simulink model "dualArrayTestComplete_noTrigger"  (R2012b)
settings: Solver=FixedStepDiscrete  StartTime=0.0  StopTime=inf  FixedStep=0.001  RelTol=1e-3
settings Model: ExplicitPartitioning=on  Creator=gilja  LastModifiedBy=NPTL
settings SolverCC: EnableConcurrentExecution=on  ConcurrentTasks=on
settings OptimizationCC: InlineParams=on  InlineInvariantSignals=on  EnhancedBackFolding=on  EfficientFloat2IntCast=on
settings HardwareCC: ProdIntDivRoundTo=Zero  ProdEndianess=LittleEndian  ProdHWDeviceType=Generic->32-bit x86 compatible
settings ModelReferenceCC: UpdateModelReferenceTargets=IfOutOfDate  ModelReferenceMinAlgLoopOccurrences=on
settings RTWCC: SystemTargetFile=xpctarget.tlc  TemplateMakefile=xpc_default_tmf  Description=xPC Target  ProcessScript=xpctarget_make_rtw_hook  RTWCompilerOptimization=On
settings CodeAppCC: MaxIdLength=62
settings xpcTargetCC: TargetFcnLib=ansi_tfl_table_tmw.mat  CodeReplacementLibrary=XPC_BLAS  ParMdlRefBuildCompliant=on  ConcurrentExecutionCompliant=on  CombineSignalStateStructs=off  GRTInterface=on  xPCTaskExecutionProfile=on  xPCRL32EventNumber=5000  xPCIRQSourceBoard=Parallel_Port  xPCIOIRQSlot=0x378  xPCisDownloadable=off  xPCLoadParamSetFile=off  xPCConcurrentTasks=off  xPCEnableSFAnimation=off

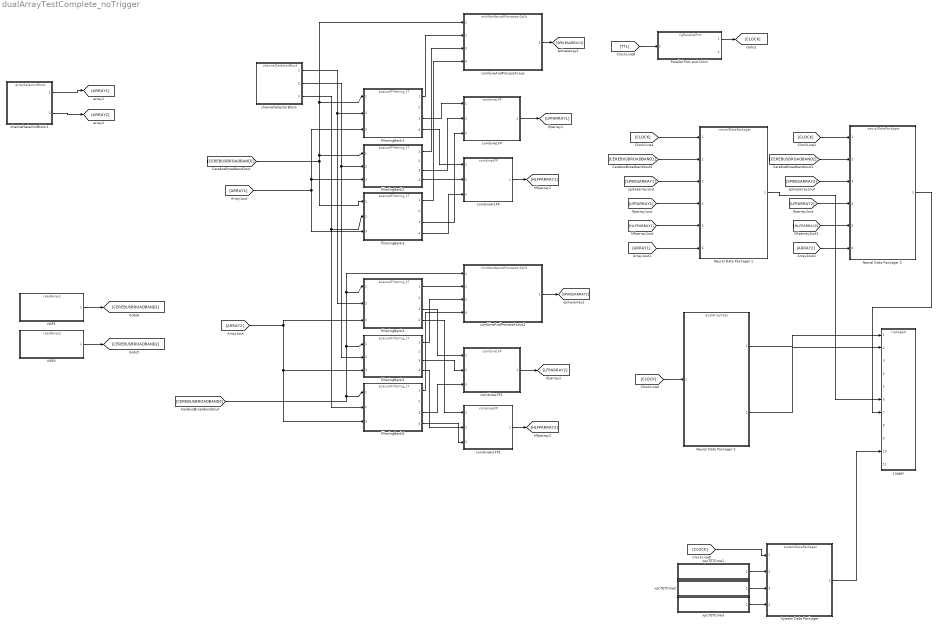
== system dualArrayTestComplete_noTrigger ==
  Logger : ModelReference  ModelNameDialog=rigLogger  SimulationMode=Normal  ModelReferenceVersion=1.134  CopyOfModelName=rigLogger  DefaultDataLogging=on
  NSP1 : ModelReference  ModelNameDialog=readArray1  SimulationMode=Normal  ModelReferenceVersion=1.97  CopyOfModelName=readArray1  DefaultDataLogging=on
  NSP2 : ModelReference  ModelNameDialog=readArray2  SimulationMode=Normal  ModelReferenceVersion=1.98  CopyOfModelName=readArray2  DefaultDataLogging=on
  Neural Data Packager 1 : ModelReference  ModelNameDialog=neuralDataPackager  SimulationMode=Normal  ModelReferenceVersion=1.161  CopyOfModelName=neuralDataPackager  DefaultDataLogging=on
  Neural Data Packager 2 : ModelReference  ModelNameDialog=neuralDataPackager  SimulationMode=Normal  ModelReferenceVersion=1.161  CopyOfModelName=neuralDataPackager  DefaultDataLogging=on
  Neural Data Packager 3 : ModelReference  ModelNameDialog=dualArrayTask  SimulationMode=Normal  ModelReferenceVersion=1.98  CopyOfModelName=dualArrayTask  DefaultDataLogging=on
  Parallel Port and Clock : ModelReference  ModelNameDialog=rigParallelPort  SimulationMode=Normal  ModelReferenceVersion=1.93  CopyOfModelName=rigParallelPort  DefaultDataLogging=on
  System Data Packager : ModelReference  Priority=0  ModelNameDialog=systemDataPackager  SimulationMode=Normal  ModelReferenceVersion=1.180  CopyOfModelName=systemDataPackager  DefaultDataLogging=on
  channelSelectorBlock : ModelReference  ModelNameDialog=channelSelectorBlock  SimulationMode=Normal  ModelReferenceVersion=1.36  CopyOfModelName=channelSelectorBlock  DefaultDataLogging=on
  channelSelectorBlock1 : ModelReference  ModelNameDialog=arraySelectorBlock  SimulationMode=Normal  ModelReferenceVersion=1.40  CopyOfModelName=arraySelectorBlock  DefaultDataLogging=on
  combineAndProcessAcaus : ModelReference  ModelNameDialog=minMaxNeuralProcessorSplit  SimulationMode=Normal  ModelReferenceVersion=1.34  CopyOfModelName=minMaxNeuralProcessorSplit  DefaultDataLogging=on
  combineAndProcessAcaus1 : ModelReference  ModelNameDialog=minMaxNeuralProcessorSplit  SimulationMode=Normal  ModelReferenceVersion=1.34  CopyOfModelName=minMaxNeuralProcessorSplit  DefaultDataLogging=on
  combineHLFP : ModelReference  ModelNameDialog=combineLFP  SimulationMode=Normal  ModelReferenceVersion=1.38  CopyOfModelName=combineLFP  DefaultDataLogging=on
  combineHLFP1 : ModelReference  ModelNameDialog=combineLFP  SimulationMode=Normal  ModelReferenceVersion=1.38  CopyOfModelName=combineLFP  DefaultDataLogging=on
  combineLFP : ModelReference  ModelNameDialog=combineLFP  SimulationMode=Normal  ModelReferenceVersion=1.38  CopyOfModelName=combineLFP  DefaultDataLogging=on
  combineLFP1 : ModelReference  ModelNameDialog=combineLFP  SimulationMode=Normal  ModelReferenceVersion=1.38  CopyOfModelName=combineLFP  DefaultDataLogging=on
  filteringBank{1..6} (6 alike) : ModelReference  ModelNameDialog=acausalFiltering_t7  SimulationMode=Normal  ModelReferenceVersion=1.72  CopyOfModelName=acausalFiltering_t7  DefaultDataLogging=on
  xpcTETCore1 : ModelReference  Priority=0  ModelNameDialog=xpcTETMulticore  SimulationMode=Normal  ModelReferenceVersion=1.188  CopyOfModelName=xpcTETMulticore  DefaultDataLogging=on
  xpcTETCore2 : ModelReference  Priority=0  ModelNameDialog=xpcTETMulticore  SimulationMode=Normal  ModelReferenceVersion=1.188  CopyOfModelName=xpcTETMulticore  DefaultDataLogging=on
  xpcTETCore3 : ModelReference  Priority=0  ModelNameDialog=xpcTETMulticore  SimulationMode=Normal  ModelReferenceVersion=1.188  CopyOfModelName=xpcTETMulticore  DefaultDataLogging=on
  wires:
  filteringBank1/1 -> combineAndProcessAcaus/2
  channelSelectorBlock/1 -> filteringBank4/2, filteringBank1/2
  channelSelectorBlock/2 -> filteringBank5/2, filteringBank2/2
  filteringBank2/1 -> combineAndProcessAcaus/3
  channelSelectorBlock/3 -> filteringBank6/2, filteringBank3/2
  filteringBank3/1 -> combineAndProcessAcaus/4
  filteringBank1/4 -> combineHLFP/1
  filteringBank2/4 -> combineHLFP/2
  filteringBank3/4 -> combineHLFP/3
  [SPIKESARRAY1] -> Neural Data Packager 1/3
  Neural Data Packager 1/1 -> Logger/6
  filteringBank1/3 -> combineLFP/1
  filteringBank2/3 -> combineLFP/2
  filteringBank3/3 -> combineLFP/3
  [CEREBUSBROADBAND1] -> filteringBank3/1, filteringBank2/1, combineAndProcessAcaus/1, filteringBank1/1
  [CEREBUSBROADBAND2] -> filteringBank6/1, filteringBank5/1, filteringBank4/1, combineAndProcessAcaus1/1
  filteringBank4/3 -> combineLFP1/1
  filteringBank5/3 -> combineLFP1/2
  filteringBank5/4 -> combineHLFP1/2
  filteringBank6/3 -> combineLFP1/3
  filteringBank4/4 -> combineHLFP1/1
  filteringBank6/4 -> combineHLFP1/3
  filteringBank4/1 -> combineAndProcessAcaus1/2
  filteringBank5/1 -> combineAndProcessAcaus1/3
  filteringBank6/1 -> combineAndProcessAcaus1/4
  Neural Data Packager 2/1 -> Logger/7
  [ARRAY1] -> filteringBank2/3, filteringBank1/3, filteringBank3/3
  [ARRAY2] -> filteringBank4/3, filteringBank6/3, filteringBank5/3
  Parallel Port and Clock/1 -> [CLOCK]
  [CLOCK] -> Neural Data Packager 2/1
  [CLOCK] -> Neural Data Packager 1/1
  combineHLFP/1 -> [HLFPARRAY1]
  [HLFPARRAY1] -> Neural Data Packager 1/5
  combineHLFP1/1 -> [HLFPARRAY2]
  [HLFPARRAY2] -> Neural Data Packager 2/5
  combineAndProcessAcaus1/1 -> [SPIKESARRAY2]
  [SPIKESARRAY2] -> Neural Data Packager 2/3
  combineAndProcessAcaus/1 -> [SPIKESARRAY1]
  combineLFP/1 -> [LFPARRAY1]
  [LFPARRAY1] -> Neural Data Packager 1/4
  combineLFP1/1 -> [LFPARRAY2]
  [LFPARRAY2] -> Neural Data Packager 2/4
  [CEREBUSBROADBAND1] -> Neural Data Packager 1/2
  [CEREBUSBROADBAND2] -> Neural Data Packager 2/2
  channelSelectorBlock1/1 -> [ARRAY1]
  channelSelectorBlock1/2 -> [ARRAY2]
  [ARRAY2] -> Neural Data Packager 2/6
  [ARRAY1] -> Neural Data Packager 1/6
  NSP1/1 -> [CEREBUSBROADBAND1]
  [TTL] -> Parallel Port and Clock/1
  NSP2/1 -> [CEREBUSBROADBAND2]
  [CLOCK] -> System Data Packager/1
  System Data Packager/1 -> Logger/10
  xpcTETCore1/1 -> System Data Packager/2
  xpcTETCore2/1 -> System Data Packager/3
  xpcTETCore3/1 -> System Data Packager/4
  [CLOCK] -> Neural Data Packager 3/1
  Neural Data Packager 3/1 -> Logger/1
  Neural Data Packager 3/2 -> Logger/2
